simulink model "Semi_Active_System_Model"  (R2024a)
settings: Solver=VariableStepAuto  StartTime=0.0  StopTime=40  RelTol=1e-3
settings Model: SimulationMode=accelerator  Creator=LENOVO  LastModifiedBy=Jashwanth
settings SolverCC: AlgebraicLoopSolver=TrustRegion
settings DataIOCC: ReturnWorkspaceOutputs=off
settings DebuggingCC: MaxConsecutiveZCsMsg=none  UnconnectedInputMsg=warning  UnconnectedOutputMsg=warning  UnconnectedLineMsg=warning  ArithmeticOperatorsInVariantConditions=warning
settings ModelReferenceCC: EnableRefExpFcnMdlSchedulingChecks=on
settings SFSimCC: SimUseLocalCustomCode=off  CustomCodeUndefinedFunction=UseInterfaceOnly
settings RTWCC: RTWUseLocalCustomCode=off  GPUComputeCapability=3.5

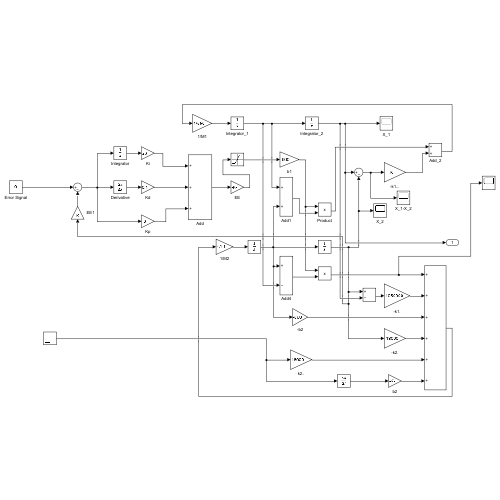
[thumbnail: Simulink's stored preview of the top-level diagram]
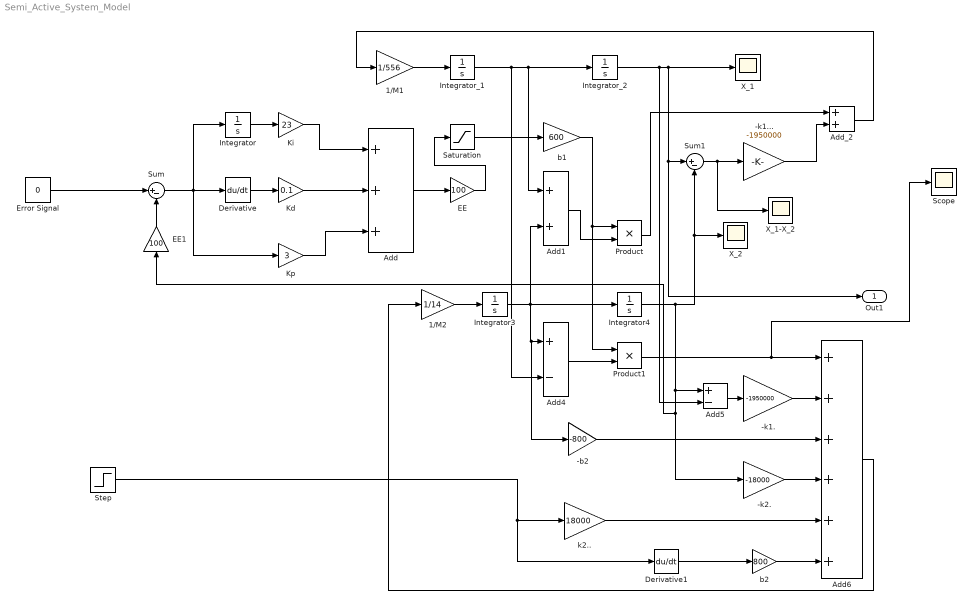
== system Semi_Active_System_Model ==
  -b2 : Gain  Gain=-800
  -k1. : Gain  Gain=-1950000
  -k1... : Gain  Gain=-1950000
  -k2. : Gain  Gain=-18000
  1/M1 : Gain  Gain=1/556
  1/M2 : Gain  Gain=1/14
  "Add " : Sum  Inputs=+++
  "Add1 " : Sum
  "Add4 " : Sum  Inputs=+-
  Add5 : Sum  Inputs=+-
  Add6 : Sum  Inputs=++++++
  Add_2 : Sum
  "Derivative " : Derivative
  Derivative1 : Derivative
  EE : Gain  Gain=100
  EE1 : Gain  Gain=100
  Error Signal : Constant  Value=0
  "Integrator " : Integrator
  Integrator3 : Integrator
  Integrator4 : Integrator
  "Integrator_1 " : Integrator
  "Integrator_2 " : Integrator
  Kd : Gain  Gain=0.1
  Ki : Gain  Gain=23
  Kp : Gain  Gain=3
  "Product " : Product
  Product1 : Product
  Saturation : Saturate  UpperLimit=1  LowerLimit=-1
  Scope : Scope
  Step : Step  Time=5  SampleTime=0
  Sum : Sum  Inputs=|+-
  Sum1 : Sum  Inputs=|+-
  X_1 : Scope
  X_1-X_2 : Scope
  X_2 : Scope
  b1 : Gain  Gain=600
  b2 : Gain  Gain=800
  k2.. : Gain  Gain=18000
  Out1 : Outport  VectorParamsAs1DForOutWhenUnconnected=off
  wires:
  "Integrator "/1 -> Ki/1
  "Derivative "/1 -> Kd/1
  Kp/1 -> "Add "/3
  Kd/1 -> "Add "/2
  Ki/1 -> "Add "/1
  Sum/1 -> Kp/1, "Integrator "/1, "Derivative "/1
  "Add "/1 -> EE/1
  EE/1 -> Saturation/1
  Saturation/1 -> b1/1
  1/M1/1 -> "Integrator_1 "/1
  "Integrator_1 "/1 -> "Add4 "/2, "Add1 "/1, "Integrator_2 "/1
  "Integrator_2 "/1 -> Add5/2, X_1/1, Sum1/1, Out1/1
  -k1.../1 -> Add_2/2
  Sum1/1 -> -k1.../1, X_1-X_2/1
  1/M2/1 -> Integrator3/1
  Integrator4/1 -> X_2/1, Sum1/2, Add5/1, EE1/1, -k2./1
  Integrator3/1 -> "Add1 "/2, Integrator4/1, -b2/1, "Add4 "/1
  "Add4 "/1 -> Product1/2
  b1/1 -> "Product "/1, Product1/1
  Add_2/1 -> 1/M1/1
  Product1/1 -> Scope/1, Add6/1
  -k1./1 -> Add6/2
  Add5/1 -> -k1./1
  -k2./1 -> Add6/4
  -b2/1 -> Add6/3
  "Add1 "/1 -> "Product "/2
  Derivative1/1 -> b2/1
  b2/1 -> Add6/6
  k2../1 -> Add6/5
  Step/1 -> k2../1, Derivative1/1
  "Product "/1 -> Add_2/1
  Add6/1 -> 1/M2/1
  Error Signal/1 -> Sum/1
  EE1/1 -> Sum/2
